simulink subsystem "caravan_battery_modell"  (R2023a)
settings: Solver=VariableStepAuto  StartTime=0.0  StopTime=10.0  RelTol=1e-3
undefined symbols (not defined in the file or in its folder): Ion, Lithium, powergui, sps_lib
libraries: spsControlledCurrentSourceLib x1, spsBatteryLib x1, eeGeneralControl x1
settings Model: Creator=sandu  LastModifiedBy=sandu

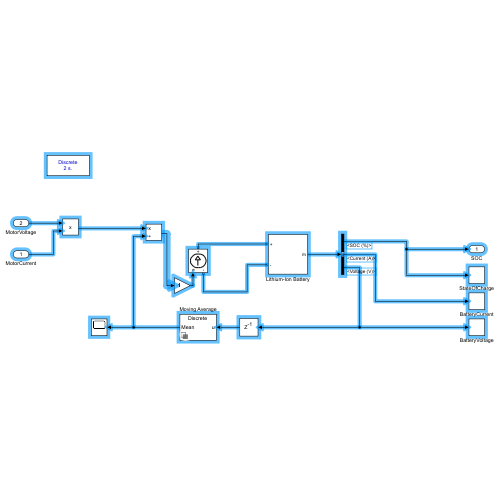
[thumbnail: Simulink's stored preview of the top-level diagram]
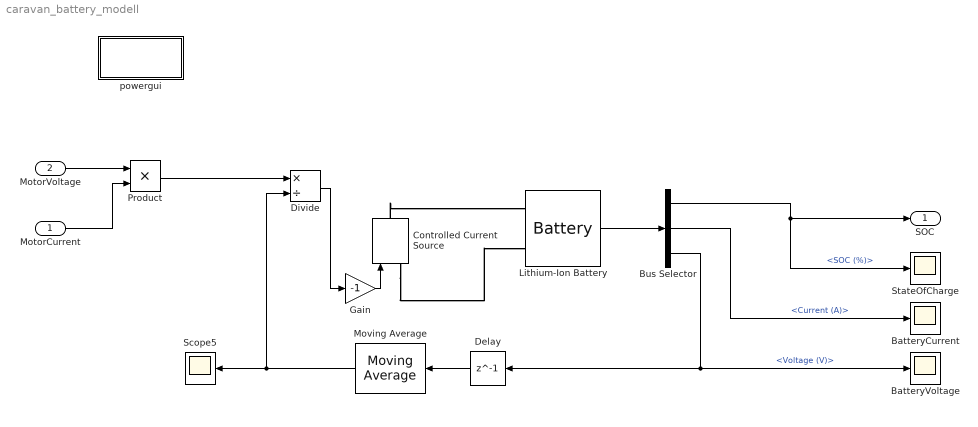
== system caravan_battery_modell ==
  MotorCurrent : Inport
  MotorVoltage : Inport  Port=2
  BatteryCurrent : Scope
  BatteryVoltage : Scope
  Bus Selector : BusSelector  OutputSignals=SOC (%),Current (A),Voltage (V)
  Controlled Current Source : spsControlledCurrentSourceLib/Controlled Current Source  Initialize=on  Source_Type=AC  Amplitude=0  Phase=0  Frequency=0  Measurements=None
  Delay : Delay  DelayLength=1  InitialCondition=0
  Divide : Product  Inputs=*/
  Gain : Gain  Gain=-1
  Lithium-Ion Battery : spsBatteryLib/Battery  BatType=Lithium-Ion  ShowTempParam=off  ThermalPreset=no  ShowAgeParam=on  NomV=370  NomQ=300  SOC=100  Batt_Tr=0.1  PresetModel=on  MaxQ=300  MinV=277.5  FullV=430.6752  Dis_rate=130.4348  R=0.012333  Normal_OP=271.3043  expZone="[399.7428      14.73913]"  current=[1.2 0.6 0.3]  Units=Time  Tci=20  NomT=25  T2=0  MaxQ2=2.208  FullV2=3.45  Normal_OP2=2.8  expZone2="[3.22        0.23]"  Rca=0.6  ti=1000  Dp=0  Neq0=0  Tsim=1e6  Ta1=25  Qeol=5.4*0.9  Reol=0.013333*1.2  Char_age=[2.3478, 3]  Dis_age=[2.3478, 10]  N1=1500  N2=10500  N3=1000  N4=1400  Ta2=45  N5=950
      settings: LibrarySourceBlock=electricdrivelib/Extra Sources/Battery
  Moving Average : eeGeneralControl/Moving Average  VariantControl=Variant1  LabelModeActiveChoice=Discrete  f=0.01  x0=420  BufferSize=8192  Ts=-1
      settings: LibrarySourceBlock=ee_sl_lib/General Control/Moving Average
  Product : Product
  Scope5 : Scope
  StateOfCharge : Scope
  powergui : Subsystem  Priority=1  AncestorBlock=sps_lib/powergui  DialogController=POWERSYS.PowerSysDialog  InitFcn=powergui( 'InitFcn_Callback' , gcb , 0 , [ ] );  mask(PSB option menu block){SimulationMode=Discrete, SampleTime=2, frequency=60, Iterations=50, frequencyindice=0, Pbase=100e6, ErrMax=1e-4, UnitsV=kV, UnitsW=MW, buscounter=0, FunctionMessages=off, echomessages=off, EnableUseOfTLC=off, CurrentSourceSwitches=off, DisableSnubberDevices=off, DisableRonSwitches=off, DisableVfSwitches=off, DisplayEquations=off, AutomaticDiscreteSolvers=off, SolverType=Tustin/Backward Euler (TBE), Interpol=off, ExternalGateDelay=off, methode=off, Ts=100, x0status=blocks, SPID=on, SwTol=0, HookPort=off, NonlinearTolerance=1e-4, nMaxIteration=100, ContinueOnMaxIteration=off, RestoreLinks=warning, ResistiveCurrentMeasurement=off, Frange=[0:2:500], Ylog=off, Xlog=on, ShowGrid=off, save=off, variable=ZData, structure=0, ZoomFFT=off, StartTime=0.0, cycles=1, DisplayStyle=1, fundamental=60, FreqAxis=off, MaxFrequency=1000, frequencyindicesteady=1, RmsSteady=1, display=off}
      mask prompts: SimulationMode "Simulation type:"; SampleTime "Sample time (s):"; frequency "Frequency (Hz):"; Iterations "Max iterations"; frequencyindice "Frequency (Hz)"; Pbase "Base power (VA)"; ErrMax "PQ tolerance (pu)"; UnitsV "Voltage units"; UnitsW "Power units"; buscounter "Load flow bus counter"; FunctionMessages "Disable Specialized Power Systems warnings"; echomessages "Display Specialized Power Systems compilation messages"; EnableUseOfTLC "Use TLC file when in Accelerator Simulation Mode and for code generation"; CurrentSourceSwitches "Disable ideal switching"; DisableSnubberDevices "Disable snubbers in switching devices"; DisableRonSwitches "Disable Ron resistances in switching devices"; DisableVfSwitches "Disable forward voltages in switching devices"; DisplayEquations "Display circuit differential equations"; AutomaticDiscreteSolvers "Automatically handle Discrete solver and Advanced tab solver settings of blocks"; SolverType "Discrete solver"; Interpol "Interpolate switching events"; ExternalGateDelay "Use time-stamped gate signals"; methode "Store switching topologies"; Ts "Buffer size (MBytes):"; x0status "Start simulation with initial electrical states from:"; SPID "Use ideal switching devices"; SwTol "Switch tolerance"; HookPort "Allow multiple powergui blocks"; NonlinearTolerance "Solver tolerance"; nMaxIteration "Maximum number of iterations"; ContinueOnMaxIteration "Continue Simulation if maximum number of iterations is reached"; RestoreLinks "Restore disabled links of Simscape Power Systems ST blocks:"; ResistiveCurrentMeasurement "Use non ideal current measurement blocks (1e-4Ohm internal resistance)"; Frange "Frequency Range"; Ylog "Log impedance"; Xlog "log Frequency"; ShowGrid "grid"; save "Save Data To Workspace"; variable "Variable Name"; structure "Structure Name (PSBFFTSCOPE)"; ZoomFFT "ZoomFFT (PSBFFTSCOPE)"; StartTime "Start Time (PSBFFTSCOPE)"; cycles "Cycles (PSBFFTSCOPE)"; DisplayStyle "Display style (PSBFFTSCOPE)"; fundamental "Fundamental (PSBFFTSCOPE)"; FreqAxis "Frequency Axis (PSBFFTSCOPE)"; MaxFrequency "Max Frequency (PSBFFTSCOPE)"; frequencyindicesteady "Frequency indice (STEADYSTATE)"; RmsSteady "RMS display (STEADYSTATE)"; display "Display Results"
      mask help: Set simulation type, simulation parameters, and preferences.
      mask init:
      | dispMessage = '';
      | dispMessage = powergui('MaskInitialization',gcb,SimulationMode,SampleTime);
      settings: LibrarySourceBlock=sps_lib/powergui  PreSaveFcn=powergui( 'PreSaveFcn_Callback' , gcb , [ ] , [ ] );  OpenFcn=sps_rtmsupport('OpenFcn',gcbh)
      mask Help: helpview(psbhelp)
      mask TypeOptions SimulationMode: Continuous | Discrete | Phasor | Discrete phasor
      mask Callback SimulationMode: powergui('SimulationType',[],[],gcb);
      mask TypeOptions UnitsV: V | kV
      mask TypeOptions UnitsW: W | kW | MW
      mask Callback CurrentSourceSwitches: powergui('SimulationType',[],[],gcb);
      mask Callback AutomaticDiscreteSolvers: powergui('SimulationType',[],[],gcb);
      mask TypeOptions SolverType: Tustin/Backward Euler (TBE) | Tustin | Backward Euler
      mask Callback SolverType: powergui('SimulationType',[],[],gcb);
      mask Callback Interpol: powergui('SimulationType',[],[],gcb);
      mask Callback ExternalGateDelay: powergui('SimulationType',[],[],gcb);
      mask Callback methode: powergui('SimulationType',[],[],gcb);
      mask TypeOptions x0status: blocks | steady | zero
      mask TypeOptions RestoreLinks: yes | warning | no
      mask Callback display: sps_rtmsupport('parametereditingmodes',gcbh) % Will be executed last in parameter callbacks to ensure mask enable consistency
      mask DialogControl SolverTab Prompt: Solver
      mask DialogControl AutoSolverNote Prompt: The Simulation type parameter is governed by Simulink. To access the Powergui solver settings, unselect auto (Automatic solver selection) solver in the Simulink solver options.
      mask DialogControl Apps Prompt: Apps
      mask DialogControl StateAnalyzer Prompt: Measurements and States Analyzer
      mask DialogControl StateAnalyzer Callback: powerStates(bdroot(gcb))
      mask DialogControl LineParameterCalculator Prompt: Line Parameter Calculator
      mask DialogControl LineParameterCalculator Callback:
      | close_system(gcb)
      | powerLineParameters
      mask DialogControl CableParameterCalculator Prompt: Cable Parameter Calculator
      mask DialogControl CableParameterCalculator Callback:
      | close_system(gcb)
      | powerCableParameters
      mask DialogControl LineDecoupler Prompt: Line Decoupler
      mask DialogControl LineDecoupler Tooltip: Click to replace selected Distributed Parameters Line blocks with Decoupling Line blocks
      mask DialogControl LineDecoupler Callback:
      | close_system(gcb);
      | DecouplingLineReplace(gcs)
      mask DialogControl LoadFlowAnalyzer Prompt: Load Flow Analyzer
      mask DialogControl LoadFlowAnalyzer Callback:
      | close_system(gcb)
      | powerLoadFlow
      mask DialogControl LoadFlowParameters Prompt: Load Flow Parameters
      mask DialogControl ImpedanceCalculator Prompt: Impedance Calculator
      mask DialogControl ImpedanceCalculator Callback:
      | close_system(gcb);
      | powerImpedance(bdroot(gcs));
      mask DialogControl FFTAnalyzer Prompt: FFT Analyzer
      mask DialogControl FFTAnalyzer Callback:
      | close_system(gcb)
      | power_fftscope(bdroot(gcb),gcb)
      mask DialogControl LinearSystemAnalyzer Prompt: Linear System Analyzer
      mask DialogControl LinearSystemAnalyzer Callback:
      | close_system(gcb)
      | power_ltiview(bdroot(gcb))
      mask DialogControl HysteresisDesigner Prompt: Hysteresis Designer
      mask DialogControl HysteresisDesigner Callback:
      | close_system(gcb)
      | powerHysteresis('hysteresis.mat')
      mask DialogControl BlockCustomizer Prompt: Block Customizer
      mask DialogControl BlockCustomizer Callback:
      | close_system(gcb);
      | power_customize;
      mask DialogControl ReportGenerator Prompt: Report Generator
      mask DialogControl ReportGenerator Callback:
      | close_system(gcb)
      | power_report(bdroot(gcb))
      mask DialogControl obsolete Prompt: ...
      mask DialogControl MachineInitialization Prompt: Machine Initialization
      mask DialogControl MachineInitialization Callback:
      | close_system(gcb)
      | powericon('machineInitTool',bdroot(gcb),gcb)
      mask DialogControl Preferences Prompt: Preferences
      mask DialogControl Solver Prompt: Solver
      mask DialogControl SolverDetails Prompt: Solver details for nonlinear elements
      mask Display: color('blue'),disp(dispMessage)
  SOC : Outport
  wires:
  Gain/1 -> Controlled Current Source/1
  MotorVoltage/1 -> Product/1
  Lithium-Ion Battery/1 -> Bus Selector/1
  MotorCurrent/1 -> Product/2
  Delay/1 -> Moving Average/1
  Product/1 -> Divide/1
  Bus Selector/1 -> SOC/1, StateOfCharge/1  "<SOC (%)>"
  Bus Selector/3 -> Delay/1, BatteryVoltage/1  "<Voltage (V)>"
  Moving Average/1 -> Divide/2, Scope5/1
  Bus Selector/2 -> BatteryCurrent/1  "<Current (A)>"
  Divide/1 -> Gain/1
  connections:
  Controlled Current Source/RConn1 -- Lithium-Ion Battery/LConn1
  Controlled Current Source/LConn1 -- Lithium-Ion Battery/LConn2

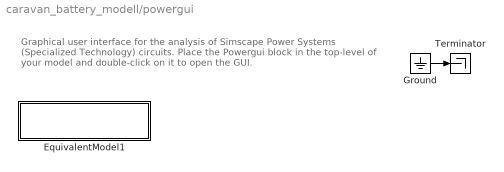
== system caravan_battery_modell/powergui ==
  note: Graphical user interface for the analysis of
      | Simscape Power Systems (Specialized Technology) circuits.
      | Place the Powergui block in the top-level of your model and double-click
      | on it to open the GUI.
  EquivalentModel1 : Subsystem
      mask init:
      | S  = GetDataForEquivalentModel('Discrete',gcbh);
      mask Display:
      | color('red')
      | disp('EQUIVALENT CIRCUIT\nDiscrete')
  Ground : Ground
  Terminator : Terminator
  wires:
  Ground/1 -> Terminator/1

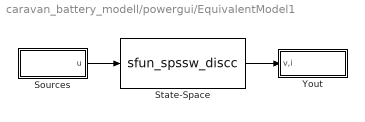
== system caravan_battery_modell/powergui/EquivalentModel1 ==
  Sources : Subsystem
  State-Space : S-Function  FunctionName=sfun_spssw_discc  Parameters=S.Ts,S.A, S.B, S.C, S.D, S.x0,S.EnableUseOfTLC  SFunctionDeploymentMode=off  EnableBusSupport=off
  Yout : Subsystem
  wires:
  Sources/1(u) -> State-Space/1
  State-Space/1 -> Yout/1(v,i)

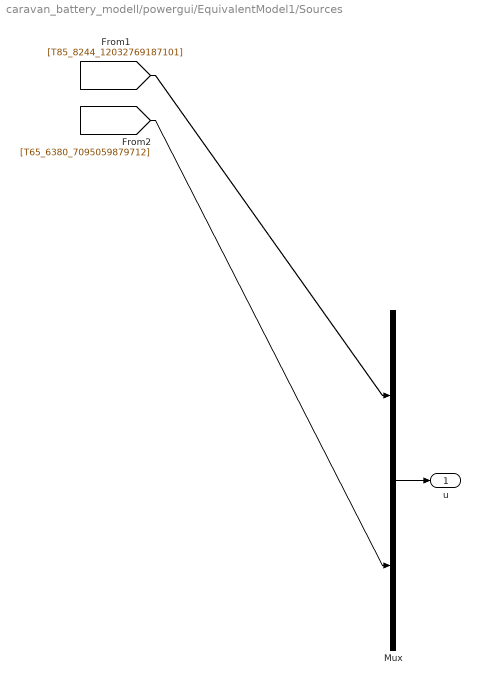
== system caravan_battery_modell/powergui/EquivalentModel1/Sources ==
  Mux : Mux  Inputs=[1 1]
  u : Outport  VectorParamsAs1DForOutWhenUnconnected=off
  wires:
  [T65_6380_7095059879712] -> Mux/2
  [T85_8244_12032769187101] -> Mux/1
  Mux/1 -> u/1

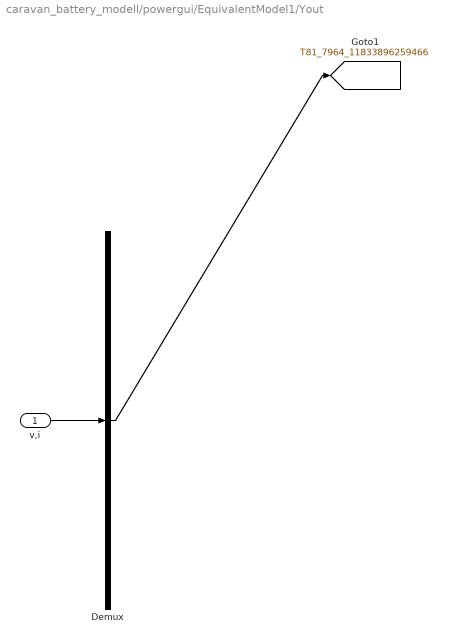
== system caravan_battery_modell/powergui/EquivalentModel1/Yout ==
  v,i : Inport
  Demux : Demux  Outputs=1
  tag scope: T81_7964_11833896259466=global
  wires:
  Demux/1 -> [T81_7964_11833896259466]
  v,i/1 -> Demux/1
